simulink model "sim_all"  (R2020a)
settings: Solver=VariableStepAuto  StartTime=0.0  StopTime=2000  RelTol=1e-3
undefined symbols (not defined in the file or in its folder): a1, a2, alpha1, alpha2, cornerA, cornerB, cornerC, cornerD, ctrl_clockwise, ctrl_int_bound_or, ctrl_int_bound_pos, ctrl_k_or, ctrl_k_pos, ctrl_Ki_vel, ctrl_Kp_v_pos, ctrl_Kp_vel, ctrl_TAM, ctrl_Ts, ctrl_va_uncontrolled, ctrl_vel_uncontrolled, D, dead_zone_limit, depth, DiscIntNeverNeededParam, distanceFromWall, initInspectedSide, initPoint, mod_A, mod_Cd_F, mod_Cd_M, mod_eta_init, mod_g, mod_h0, mod_Ixx, mod_Iyy, mod_Izz, mod_Kp_dot, mod_lat0, mod_lon0, mod_m, mod_Mq_dot, mod_ni_init, mod_Nr_dot, mod_p1, mod_p2, mod_p3, mod_p4, mod_p5, mod_p6, mod_R, mod_Rm, mod_t1, mod_t2, mod_t3, mod_t4, mod_t5, mod_t6, mod_W, mod_Xu_dot, mod_Yv_dot ... (+53)
libraries: simulink x8, cstblocks x6, simulink_extras x1
(part 2 of 6)

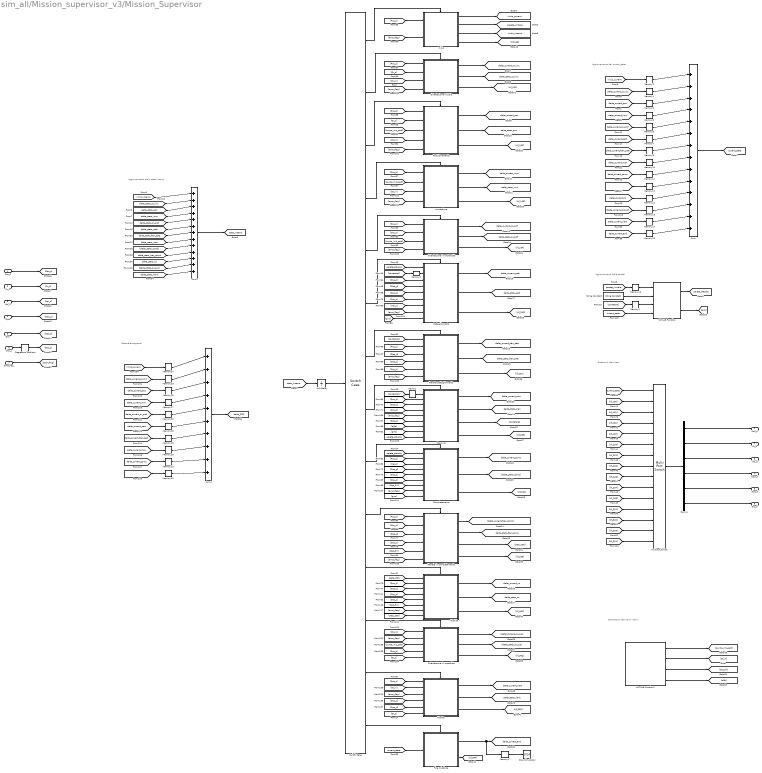
== system sim_all/Mission_supervisor_v3/Mission_Supervisor ==
  note: Gestore emergenza
  note: Generatore riferimenti interni
  note: Aggiornamento dello stato interno
  note: Aggiornamento del current_state
  note: Aggiornamento della parete
  note: Gestore di riferimenti
  Pos_S : Inport
  Or_S : Inport  Port=2
  Vel_S : Inport  Port=3
  Dpp : Inport  Port=4
  Dps : Inport  Port=5
  Orp_s : Inport  Port=6
  error_flag : Inport  Port=7
  Completamento : Subsystem  TreatAsAtomicUnit=on
  Degrees to Radians : simulink_extras/Transformations/Degrees to Radians
  Demux : Demux  Outputs=[3,3,1,1,1,1]
  Fine missione : Subsystem  TreatAsAtomicUnit=on
  Frenata in completamento : Subsystem  TreatAsAtomicUnit=on
  Frenata pattugliamento : Subsystem  TreatAsAtomicUnit=on
  Immersione : Subsystem  TreatAsAtomicUnit=on
  Inizio : Subsystem  TreatAsAtomicUnit=on
  MATLAB Function : MATLAB Function  TreatAsAtomicUnit=on
  MATLAB Function1 : MATLAB Function  TreatAsAtomicUnit=on
  Manovra : Subsystem  TreatAsAtomicUnit=on
  Memory{,1..2,4..15,17..21,25..30} (26 alike) : Memory
  Memory16 : Memory  InitialCondition=initInspectedSide
  Memory24 : Memory  InitialCondition=100
  Memory3 : Memory  InitialCondition=100
  Multiport Switch : MultiPortSwitch  DataPortOrder=Specify indices  Inputs=2  DataPortIndices={100,101,102,103,104,201,202,203,204,205,301,302,303,304}
  Orientazione Iniziale : Subsystem  TreatAsAtomicUnit=on
  Orientazione in profondità : Subsystem  TreatAsAtomicUnit=on
  Orientazione in superficie : Subsystem  TreatAsAtomicUnit=on
  Pattugliamento : Subsystem  TreatAsAtomicUnit=on
  Posizionamento : Subsystem  TreatAsAtomicUnit=on
  Rientro : Subsystem  TreatAsAtomicUnit=on
  Risalita : Subsystem  TreatAsAtomicUnit=on
  Stop Simulation : Stop
  String Constant : StringConstant  String=inspectionDirection
  Sum : Sum  Inputs=|++++++++++++++
  Sum1 : Sum  Inputs=|+++++++++++++
  Sum4 : Sum  Inputs=|++++++++++
  Switch Case : SwitchCase  CaseConditions={100,101,102,103,104,201,202,203,204,205,301,302,303,304}  ShowDefaultCase=off
  Unit Delay : UnitDelay  InitialCondition=stato  SampleTime=Ts_supervisor  HasFrameUpgradeWarning=on
  Pos_d : Outport
  Or_d : Outport  Port=2
  Vel_d : Outport  Port=3
  Dpp_d : Outport  Port=4
  Dps_d : Outport  Port=5
  Orp_d : Outport  Port=6
  tag scope: current_state=global, delta_SOS=global, delta_current_comp=global, delta_current_end=global, delta_current_fren_patt=global, delta_current_imm=global, delta_current_man=global, delta_current_or_iniz=global, delta_current_or_prof=global, delta_current_patt=global, delta_current_pos=global, delta_current_rient=global, delta_current_ris=global, delta_stato_fren_comp=global, delta_stato_fren_patt=global, delta_stato_imm=global, delta_stato_man=global, delta_stato_or_iniz=global, delta_stato_or_prof=global, delta_stato_patt=global, delta_stato_pos=global, delta_stato_rient=global, delta_stato_ris=global, inizio_current=global, inizio_interno=global, parete_attuale=global, parete_iniziale=global, stato_interno=global
  wires:
  [delta_stato_fren_comp] -> Sum1/10
  [delta_SOS] -> Risalita/1(delta_SOS)
  [delta_current_patt] -> Memory7/1
  [delta_current_pos] -> Memory5/1
  Immersione/1(delta_current_immers) -> [delta_current_imm]
  Posizionamento/3(Outport) -> [rif_102]
  Rientro/2(delta_stato_rient) -> [delta_stato_rient]
  [delta_stato_or_iniz] -> Sum1/2
  [inizio_interno] -> Sum1/1
  Memory6/1 -> Sum/4
  Orientazione Iniziale/1(delta_current_or_iniz) -> [delta_current_or_iniz]
  [delta_current_end] -> Memory15/1
  Pattugliamento/1(delta_current_patt) -> [delta_current_patt]
  Memory15/1 -> Sum/14
  Orientazione in profondità/2(delta_stato_or_prof) -> [delta_stato_or_prof]
  Memory12/1 -> Sum/10
  Memory8/1 -> Sum/7
  Completamento/3(Outport) -> [rif_204]
  Pattugliamento/2(delta_stato_patt) -> [delta_stato_patt]
  [delta_stato_man] -> Sum1/8
  Frenata in completamento/1(delta_current_fren_comp) -> [delta_current_fren_comp]
  Frenata pattugliamento/1(delta_current_fren_patt) -> [delta_current_fren_patt]
  Sum/1 -> [current_state]
  Inizio/1(current_state) -> [inizio_current]
  Memory4/1 -> Sum/2
  Posizionamento/2(delta_stato_posiz) -> [delta_stato_pos]
  [delta_stato_pos] -> Sum1/3
  Completamento/2(delta_stato_comp) -> [delta_stato_comp]
  [contatore] -> Memory2/1
  Memory17/1 -> Stop Simulation/1
  [delta_stato_imm] -> Sum1/4
  [delta_current_imm] -> Memory6/1
  [stato_interno] -> Unit Delay/1
  Sum1/1 -> [stato_interno]
  Inizio/2(parete_attuale) -> [parete_iniziale]
  [delta_stato_comp] -> Sum1/9
  [delta_stato_patt] -> Sum1/6
  Risalita/2(delta_stato_ris) -> [delta_stato_ris]
  [delta_current_fren_patt] -> Memory8/1
  [delta_current_or_prof] -> Memory9/1
  Rientro/1(delta_current_rient) -> [delta_current_rient]
  [current_state] -> Fine missione/1(current_state)
  Unit Delay/1 -> Switch Case/1
  [parete_attuale] -> Pattugliamento/1(parete)
  Memory7/1 -> Sum/6
  Orientazione in profondità/1(delta_current_or_prof) -> [delta_current_or_prof]
  Frenata in completamento/2(delta_stato_fren_comp) -> [delta_stato_fren_comp]
  [contatore] -> Frenata pattugliamento/1(contatore)
  Manovra/1(delta_current_man) -> [delta_current_man]
  [delta_current_fren_comp] -> Memory12/1
  Fine missione/1(delta_current_end) -> [delta_current_end], Memory17/1
  [inizio_current] -> Memory3/1
  [parete_attuale] -> Completamento/1(parete)
  Memory3/1 -> Sum/1
  Risalita/1(delta_current_ris) -> [delta_current_ris]
  [delta_stato_or_prof] -> Sum1/5
  Memory2/1 -> Pattugliamento/2(contatore)
  Memory11/1 -> Sum/9
  Posizionamento/1(delta_current_posiz) -> [delta_current_pos]
  Rientro/3(Outport) -> [rif_303]
  Inizio/3(delta_stato) -> [inizio_interno]
  [delta_current_comp] -> Memory11/1
  [delta_stato_fren_patt] -> Sum1/7
  [delta_stato_ris] -> Sum1/11
  Orientazione in profondità/3(Outport) -> [rif_104]
  Frenata pattugliamento/3(Outport) -> [rif_202]
  Orientazione Iniziale/2(delta_stato_or_iniz) -> [delta_stato_or_iniz]
  Fine missione/2(Outport) -> [rif_304]
  Memory10/1 -> Sum/8
  [delta_current_man] -> Memory10/1
  Immersione/2(delta_stato_immers) -> [delta_stato_imm]
  Manovra/2(delta_stato_man) -> [delta_stato_man]
  Orientazione Iniziale/3(Outport) -> [rif_101]
  [delta_current_or_iniz] -> Memory4/1
  Pattugliamento/3(Outport) -> [rif_201]
  Frenata pattugliamento/2(delta_stato_fren_patt) -> [delta_stato_fren_patt]
  Memory9/1 -> Sum/5
  Memory14/1 -> Sum/13
  Inizio/4(Outport) -> [rif_100]
  Risalita/3(Outport) -> [rif_301]
  Immersione/3(Outport) -> [rif_103]
  Memory5/1 -> Sum/3
  [Pos_s] -> Inizio/1(Pos_s)
  [Pos_s] -> Orientazione Iniziale/1(Pos_s)
  [Pos_s] -> Posizionamento/1(Pos_s)
  [Pos_s] -> Immersione/1(Pos_s)
  [Pos_s] -> Frenata pattugliamento/2(Pos_s)
  [Dpp_s] -> Frenata pattugliamento/3(Dpp_s)
  [Dps_s] -> Frenata pattugliamento/4(Dps_s)
  [Pos_s] -> Pattugliamento/3(Pos_s)
  [Dpp_s] -> Pattugliamento/4(Dpp_s)
  [Dps_s] -> Pattugliamento/5(Dps_s)
  [Orp_s] -> Pattugliamento/6(Orp_s)
  [Vel_s] -> Pattugliamento/7(Vel_s)
  [Orp_s] -> Frenata pattugliamento/5(Orp_s)
  [Dpp_s] -> Manovra/3(Dpp_s)
  [Orp_s] -> Manovra/4(Orp_s)
  [Pos_s] -> Manovra/2(Pos_s)
  [Pos_s] -> Completamento/2(Pos_s)
  [Vel_s] -> Completamento/3(Vel_s)
  [Dpp_s] -> Completamento/4(Dpp_s)
  [Dps_s] -> Completamento/5(Dps_s)
  [Orp_s] -> Completamento/6(Orp_s)
  [Pos_s] -> Frenata in completamento/1(Pos_s)
  [Orp_s] -> Frenata in completamento/2(Orp_s)
  [Dpp_s] -> Frenata in completamento/3(Dpp_s)
  [Dps_s] -> Frenata in completamento/4(Dps_s)
  [Pos_s] -> Risalita/2(Pos_s)
  [Dpp_s] -> Risalita/3(Dpp_s)
  [Pos_s] -> Rientro/1(Pos_s)
  Demux/2 -> Or_d/1
  [rif_202] -> Multiport Switch/8
  [current_state] -> Multiport Switch/1
  Demux/6 -> Orp_d/1
  Demux/3 -> Vel_d/1
  Multiport Switch/1 -> Demux/1
  [rif_301] -> Multiport Switch/12
  Demux/4 -> Dpp_d/1
  [rif_102] -> Multiport Switch/4
  [rif_203] -> Multiport Switch/9
  Demux/5 -> Dps_d/1
  Demux/1 -> Pos_d/1
  [rif_302] -> Multiport Switch/13
  [rif_201] -> Multiport Switch/7
  [rif_104] -> Multiport Switch/6
  [rif_205] -> Multiport Switch/11
  [rif_204] -> Multiport Switch/10
  [rif_101] -> Multiport Switch/3
  [rif_303] -> Multiport Switch/14
  [rif_103] -> Multiport Switch/5
  Completamento/1(delta_current_comp) -> [delta_current_comp]
  [Pos_s] -> Orientazione in profondità/1(Pos_s)
  [Orp_s] -> Orientazione in profondità/2(Orp_s)
  [rif_100] -> Multiport Switch/2
  [Or_s] -> Orientazione Iniziale/2(Or_s)
  [Or_in] -> Orientazione Iniziale/3(Or_in)
  [Or_in] -> Posizionamento/4(Or_in)
  [punto_iniz_patt] -> Posizionamento/3(punto iniziale)
  [dps_fin] -> Frenata in completamento/5(dps_fin)
  [punto_iniz_patt] -> Immersione/2(punto_iniz_patt)
  [punto_iniz_patt] -> Orientazione in profondità/3(Punto_iniz_patt)
  [Or_s] -> Posizionamento/2(Or_s)
  [dps_fin] -> Completamento/7(Dps_fin)
  error_flag/1 -> [error_flag]
  [error_flag] -> Frenata in completamento/6(error_flag)
  [error_flag] -> Completamento/8(error_flag)
  [error_flag] -> Manovra/5(error_flag)
  [error_flag] -> Frenata pattugliamento/6(error_flag)
  [error_flag] -> Pattugliamento/8(error_flag)
  [error_flag] -> Orientazione in profondità/4(error_flag)
  [error_flag] -> Immersione/4(error_flag)
  [error_flag] -> Posizionamento/5(error_flag)
  [error_flag] -> Orientazione Iniziale/4(error_flag)
  [error_flag] -> Inizio/2(error_flag)
  MATLAB Function1/3(dps_fin) -> [dps_fin]
  MATLAB Function1/2(Or_in) -> [Or_in]
  MATLAB Function1/1(punto_iniz_patt) -> [punto_iniz_patt]
  [Or_in] -> Immersione/3(Or_in)
  [Or_in] -> Rientro/2(Or_in)
  Memory25/1 -> Sum4/2
  Sum4/1 -> [delta_SOS]
  Memory27/1 -> Sum4/4
  Memory20/1 -> Sum4/10
  [delta_current_fren_comp] -> Memory20/1
  Memory26/1 -> Sum4/3
  Memory28/1 -> Sum4/6
  [delta_current_comp] -> Memory19/1
  Memory18/1 -> Sum4/8
  [delta_current_or_prof] -> Memory30/1
  Memory30/1 -> Sum4/5
  [delta_current_or_iniz] -> Memory25/1
  [delta_current_man] -> Memory18/1
  [delta_current_fren_patt] -> Memory29/1
  [delta_current_patt] -> Memory28/1
  [inizio_current] -> Memory24/1
  [delta_current_pos] -> Memory26/1
  [delta_current_imm] -> Memory27/1
  Memory24/1 -> Sum4/1
  Memory29/1 -> Sum4/7
  Memory19/1 -> Sum4/9
  [contatore] -> Memory1/1
  [parete_iniziale] -> Memory16/1
  [current_state] -> MATLAB Function/4(current_state)
  Memory1/1 -> MATLAB Function/3(contatore)
  String Constant/1 -> MATLAB Function/2(verso)
  Memory16/1 -> MATLAB Function/1(parete_iniziale)
  MATLAB Function/1(parete) -> [parete_attuale]
  [contatore] -> Memory/1
  Memory/1 -> Manovra/1(contatore)
  [Dps_s] -> Risalita/5(Dps_s)
  [Orp_s] -> Risalita/4(Orp_s)
  [dps_fin] -> Risalita/6(Dps_fin)
  Switch Case/1 -> Inizio/Action
  Switch Case/3 -> Posizionamento/Action
  Switch Case/2 -> Orientazione Iniziale/Action
  Switch Case/4 -> Immersione/Action
  Switch Case/5 -> Orientazione in profondità/Action
  Switch Case/6 -> Pattugliamento/Action
  Switch Case/7 -> Frenata pattugliamento/Action
  Switch Case/8 -> Manovra/Action
  Switch Case/9 -> Completamento/Action
  Switch Case/10 -> Frenata in completamento/Action
  Switch Case/11 -> Risalita/Action
  Switch Case/12 -> Orientazione in superficie/Action
  Switch Case/13 -> Rientro/Action
  Switch Case/14 -> Fine missione/Action
  Orientazione in superficie/1(delta_current_or_sup) -> [delta_current_or_sup]
  Orientazione in superficie/2(delta_stato_or_sup) -> [delta_stato_or_sup]
  Orientazione in superficie/3(Outport) -> [rif_302]
  [rif_304] -> Multiport Switch/15
  [error_flag] -> Risalita/7(error_flag)
  Memory13/1 -> Sum/12
  Memory21/1 -> Sum/11
  [delta_stato_or_sup] -> Sum1/12
  [delta_stato_rient] -> Sum1/13
  [delta_current_rient] -> Memory14/1
  [delta_current_or_sup] -> Memory13/1
  [delta_current_ris] -> Memory21/1
  [error_flag] -> Rientro/3(error_flag)
  [error_flag] -> Orientazione in superficie/2(error_flag)
  [Or_in] -> Orientazione in superficie/1(Or_in)
  [punto_iniz_patt] -> Orientazione in superficie/3(punto_iniz_patt)
  [Or_s] -> Orientazione in superficie/5(Or_s)
  [Pos_s] -> Orientazione in superficie/4(Pos_s)
  [Dps_s] -> Rientro/4(Dps_s)
  [Dpp_s] -> Rientro/5(Dpp_s)
  [Dps_s] -> Manovra/6(Dps_s)
  MATLAB Function/2(giro) -> [giro]
  [giro] -> Pattugliamento/9(giro)
  [giro] -> Completamento/9(giro)
  [SOS_205] -> Risalita/8(SOS_205)
  Pos_S/1 -> [Pos_s]
  Or_S/1 -> [Or_s]
  Vel_S/1 -> [Vel_s]
  Dpp/1 -> [Dpp_s]
  Dps/1 -> [Dps_s]
  Orp_s/1 -> Degrees to Radians/1
  Degrees to Radians/1 -> [Orp_s]
  Manovra/4("  ") -> [rif_203]
  Manovra/3(contatore_out) -> [contatore]
  Frenata in completamento/3(SOS_205) -> [SOS_205]
  Frenata in completamento/4(" ") -> [rif_205]
  [Or_s] -> Rientro/6(Or_s)
  MATLAB Function1/4(alfa) -> [alfa]
  [alfa] -> Manovra/7(alfa)
  [giro] -> Manovra/8(giro)
  [parete_attuale] -> Manovra/9(parete_attuale)

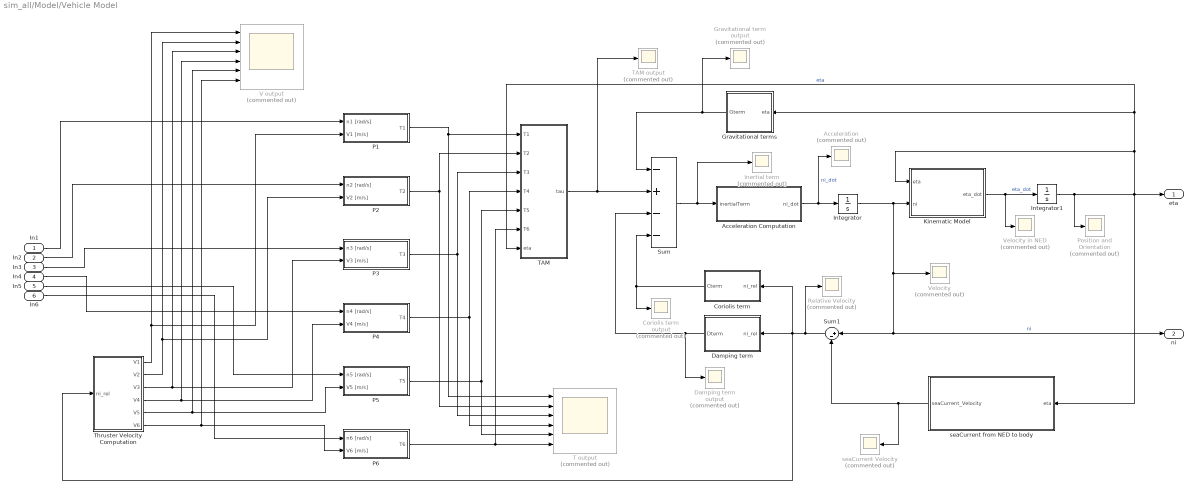
== system sim_all/Model/Vehicle Model ==
  In1 : Inport
  In2 : Inport  Port=2
  In3 : Inport  Port=3
  In4 : Inport  Port=4
  In5 : Inport  Port=5
  In6 : Inport  Port=6
  Acceleration : Scope  Commented=on
  Acceleration Computation : MATLAB Function  TreatAsAtomicUnit=on
  Coriolis term : MATLAB Function  TreatAsAtomicUnit=on
  Coriolis term output : Scope  Commented=on
  Damping term : MATLAB Function  TreatAsAtomicUnit=on
  Damping term output : Scope  Commented=on
  Gravitational term output : Scope  Commented=on
  Gravitational terms : MATLAB Function  TreatAsAtomicUnit=on
  Inertial term : Scope  Commented=on
  Integrator : Integrator  InitialCondition=mod_ni_init
  Integrator1 : Integrator  InitialCondition=mod_eta_init
  Kinematic Model : MATLAB Function  TreatAsAtomicUnit=on
  P1 : Subsystem
  P2 : Subsystem
  P3 : Subsystem
  P4 : Subsystem
  P5 : Subsystem
  P6 : Subsystem
  Position and Orientation : Scope  Commented=on
  Relative Velocity : Scope  Commented=on
  Sum : Sum  Inputs=-+--
  Sum1 : Sum  Inputs=|+-
  T output : Scope  Commented=on  NumInputPorts=6
  TAM : MATLAB Function  TreatAsAtomicUnit=on
  TAM output : Scope  Commented=on
  Thruster Velocity Computation : MATLAB Function  TreatAsAtomicUnit=on
  V output : Scope  Commented=on  NumInputPorts=6
  Velocity : Scope  Commented=on
  Velocity in NED : Scope  Commented=on
  seaCurrent Velocity : Scope  Commented=on
  seaCurrent from NED to body : MATLAB Function  TreatAsAtomicUnit=on
  eta : Outport
  ni : Outport  Port=2
  wires:
  P3/1(T3) -> TAM/3(T3), T output/3
  P5/1(T5) -> TAM/5(T5), T output/5
  P6/1(T6) -> TAM/6(T6), T output/6
  Thruster Velocity Computation/6(V6) -> P6/2(V6 [m/s]), V output/6
  Sum/1 -> Acceleration Computation/1(inertialTerm), Inertial term/1
  Integrator/1 -> Kinematic Model/2(ni), Velocity/1, ni/1, Sum1/1  "ni"
  P2/1(T2) -> TAM/2(T2), T output/2
  Acceleration Computation/1(ni_dot) -> Integrator/1, Acceleration/1  "ni_dot"
  Gravitational terms/1(Gterm) -> Sum/1, Gravitational term output/1
  P1/1(T1) -> T output/1, TAM/1(T1)
  TAM/1(tau) -> Sum/2, TAM output/1
  Thruster Velocity Computation/5(V5) -> P5/2(V5 [m/s]), V output/5
  Integrator1/1 -> Position and Orientation/1, Kinematic Model/1(eta), Gravitational terms/1(eta), TAM/7(eta), seaCurrent from NED to body/1(eta), eta/1  "eta"
  Thruster Velocity Computation/2(V2) -> V output/2, P2/2(V2 [m/s])
  Thruster Velocity Computation/1(V1) -> V output/1, P1/2(V1 [m/s])
  Damping term/1(Dterm) -> Damping term output/1, Sum/3
  Kinematic Model/1(eta_dot) -> Integrator1/1, Velocity in NED/1  "eta_dot"
  P4/1(T4) -> TAM/4(T4), T output/4
  Thruster Velocity Computation/4(V4) -> P4/2(V4 [m/s]), V output/4
  Thruster Velocity Computation/3(V3) -> P3/2(V3 [m/s]), V output/3
  Coriolis term/1(Cterm) -> Coriolis term output/1, Sum/4
  In6/1 -> P6/1(n6 [rad/s])
  In2/1 -> P2/1(n2 [rad/s])
  In5/1 -> P5/1(n5 [rad/s])
  In1/1 -> P1/1(n1 [rad/s])
  In4/1 -> P4/1(n4 [rad/s])
  In3/1 -> P3/1(n3 [rad/s])
  seaCurrent from NED to body/1(seaCurrent_Velocity) -> seaCurrent Velocity/1, Sum1/2
  Sum1/1 -> Relative Velocity/1, Thruster Velocity Computation/1(ni_rel), Damping term/1(ni_rel), Coriolis term/1(ni_rel)

== system sim_all/Navigation/Calcolo distaza pareti ==
  orient : Inport
  pos_es : Inport  Port=2
  Calcolo distanza dalle pareti : MATLAB Function  TreatAsAtomicUnit=on
  Calcolo orientazione dalla parete : MATLAB Function  TreatAsAtomicUnit=on
  dpp : Outport
  dps : Outport  Port=2
  orient_parete : Outport  Port=3
  wires:
  pos_es/1 -> Calcolo distanza dalle pareti/1(pos_es), Calcolo orientazione dalla parete/1(pos_es)
  Calcolo distanza dalle pareti/2(dps) -> dps/1
  Calcolo orientazione dalla parete/1(orient_parete) -> orient_parete/1
  orient/1 -> Calcolo orientazione dalla parete/3(orient)
  Calcolo distanza dalle pareti/1(dpp) -> dpp/1
  [parete_attuale] -> Calcolo distanza dalle pareti/2(parete_attuale), Calcolo orientazione dalla parete/2(parete_attuale)

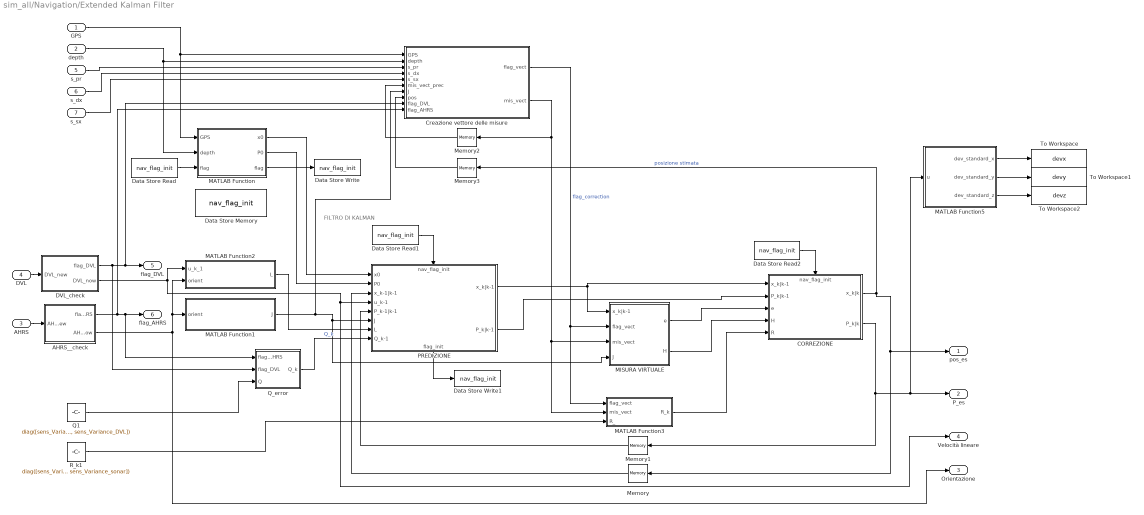
== system sim_all/Navigation/Extended Kalman Filter ==
  note: FILTRO DI KALMAN
  GPS : Inport
  depth : Inport  Port=2
  AHRS : Inport  Port=3
  DVL : Inport  Port=4
  s_pr : Inport  Port=5
  s_dx : Inport  Port=6
  s_sx : Inport  Port=7
  AHRS__check : Subsystem
  CORREZIONE : Subsystem
      settings: PortSchema="{\"entries\":[{\"content\":{\"sides\":[{\"content\":{\"connectorIds\":[\"In1\",\"In2\",\"In3\",\"In4\",\"In5\"]},\"type\":\"ConnectorPlacement.EquallySpacedRectSide\",\"uuid\":\"44d4b6e6-a4db-4e12-b0bf-41ec8347b107\"},{\"content\":{\"connectorIds\":[\"Out1\",\"Out2\"],\"side\":\"RIGHT\"},\"type\":\"ConnectorPlacement.EquallySpacedRectSide\",\"uuid\":\"9e6d7b97-2a84-49ec-a092-e75c60e4106f\"},{\"content\":{\"connectorIds\":[\"In6\"],\"side\":\"TOP\"},\"type\":\"ConnectorPlacement.EquallySpacedRectSide\",\"uuid\":\"c5d17fe6-9815-494d-a6f8-5d09015b4aeb\"}]},\"type\":\"ConnectorPlacement.EquallySpacedConnector\",\"uuid\":\"e87b91ff-8818-4035-b847-a1a4860b11e5\"}],\"packageUris\":[\"http://schema.mathworks.com/mf0/Connector/19700101\"],\"version\":\"1.0\"}"
  Creazione vettore delle misure : MATLAB Function  TreatAsAtomicUnit=on  SystemSampleTime=nav_DT
  DVL_check : Subsystem
  Data Store Memory : DataStoreMemory  DataStoreName=nav_flag_init  ShowAdditionalParam=off
  Data Store Read : DataStoreRead  DataStoreName=nav_flag_init  DataStoreElements=nav_flag_init
  Data Store Read1 : DataStoreRead  DataStoreName=nav_flag_init  DataStoreElements=nav_flag_init
  Data Store Read2 : DataStoreRead  DataStoreName=nav_flag_init  DataStoreElements=nav_flag_init
  Data Store Write : DataStoreWrite  DataStoreName=nav_flag_init  DataStoreElements=nav_flag_init
  Data Store Write1 : DataStoreWrite  DataStoreName=nav_flag_init  DataStoreElements=nav_flag_init
  MATLAB Function : MATLAB Function  TreatAsAtomicUnit=on
  MATLAB Function1 : MATLAB Function  TreatAsAtomicUnit=on
  MATLAB Function2 : MATLAB Function  TreatAsAtomicUnit=on
  MATLAB Function3 : MATLAB Function  TreatAsAtomicUnit=on  SystemSampleTime=nav_DT
  MATLAB Function5 : MATLAB Function  TreatAsAtomicUnit=on
  MISURA VIRTUALE : Subsystem
  Memory{,1..3} (4 alike) : Memory
  PREDIZIONE : Subsystem
      settings: PortSchema="{\"entries\":[{\"content\":{\"sides\":[{\"content\":{\"connectorIds\":[\"In1\",\"In2\",\"In3\",\"In4\",\"In5\",\"In6\",\"In7\",\"In8\"]},\"type\":\"ConnectorPlacement.EquallySpacedRectSide\",\"uuid\":\"afcfc03b-4c18-49df-ab20-1356d76b0e63\"},{\"content\":{\"connectorIds\":[\"Out1\",\"Out2\"],\"side\":\"RIGHT\"},\"type\":\"ConnectorPlacement.EquallySpacedRectSide\",\"uuid\":\"f068ce64-2e14-41bc-9570-b9ba38e252ee\"},{\"content\":{\"connectorIds\":[\"In9\"],\"side\":\"TOP\"},\"type\":\"ConnectorPlacement.EquallySpacedRectSide\",\"uuid\":\"07751979-165e-45fb-8dea-4cc1ad3e58f3\"},{\"content\":{\"connectorIds\":[\"Out3\"],\"side\":\"BOTTOM\"},\"type\":\"ConnectorPlacement.EquallySpacedRectSide\",\"uuid\":\"3c36a795-b00b-49e7-8b71-9706a2c2134a\"}]},\"type\":\"ConnectorPlacement.EquallySpacedConnector\",\"uuid\":\"bde89349-47ff-4cbc-a848-02c48716c9c8\"}],\"packageUris\":[\"http://schema.mathworks.com/mf0/Connector/19700101\"],\"version\":\"1.0\"}"
  Q1 : Constant  Value=diag([sens_Variance_AHRS_roll, sens_Variance_AHRS_pitch, sens_Variance_AHRS_yaw, sens_Variance_DVL, sens_Variance_DVL, sens_Variance_DVL])  VectorParams1D=off
  Q_error : Subsystem
  R_k1 : Constant  Value=diag([sens_Variance_GPS, sens_Variance_GPS, sens_Variance_depth1, sens_Variance_sonar, sens_Variance_sonar, sens_Variance_sonar])  VectorParams1D=off
  To Workspace : ToWorkspace  VariableName=devx  SaveFormat=Timeseries  SampleTime=-1
  To Workspace1 : ToWorkspace  VariableName=devy  SaveFormat=Timeseries  SampleTime=-1
  To Workspace2 : ToWorkspace  VariableName=devz  SaveFormat=Timeseries  SampleTime=-1
  pos_es : Outport
  P_es : Outport  Port=2
  Orientazione : Outport  Port=3
  Velocità lineare : Outport  Port=4
  flag_DVL : Outport  Port=5
  flag_AHRS : Outport  Port=6
  wires:
  PREDIZIONE/1(x_k|k-1) -> CORREZIONE/1(x_k|k-1), MISURA VIRTUALE/1(x_k|k-1)
  PREDIZIONE/2(P_k|k-1) -> CORREZIONE/2(P_k|k-1)
  Memory/1 -> PREDIZIONE/3(x_k-1|k-1)
  CORREZIONE/2(P_k|k) -> Memory1/1, P_es/1, MATLAB Function5/1(u)
  Memory1/1 -> PREDIZIONE/5(P_k-1|k-1)
  MISURA VIRTUALE/2(H) -> CORREZIONE/4(H)
  MISURA VIRTUALE/1(e) -> CORREZIONE/3(e)
  GPS/1 -> MATLAB Function/1(GPS), Creazione vettore delle misure/1(GPS)
  depth/1 -> MATLAB Function/2(depth), Creazione vettore delle misure/2(depth)
  s_pr/1 -> Creazione vettore delle misure/3(s_pr)
  Creazione vettore delle misure/2(mis_vect) -> MATLAB Function3/2(mis_vect), MISURA VIRTUALE/3(mis_vect), Memory2/1
  Memory2/1 -> Creazione vettore delle misure/6(mis_vect_prec)
  Creazione vettore delle misure/1(flag_vect) -> MATLAB Function3/1(flag_vect), MISURA VIRTUALE/2(flag_vect)  "flag_correction"
  s_dx/1 -> Creazione vettore delle misure/4(s_dx)
  s_sx/1 -> Creazione vettore delle misure/5(s_sx)
  MATLAB Function/2(P0) -> PREDIZIONE/2(P0)
  MATLAB Function/1(x0) -> PREDIZIONE/1(x0)
  MATLAB Function1/1(J) -> Creazione vettore delle misure/7(J), MISURA VIRTUALE/4(J), PREDIZIONE/6(J)
  MATLAB Function2/1(L) -> PREDIZIONE/7(L)
  Data Store Read/1 -> MATLAB Function/3("flag ")
  MATLAB Function/3(flag) -> Data Store Write/1
  Data Store Read1/1 -> PREDIZIONE/9(nav_flag_init)
  Data Store Read2/1 -> CORREZIONE/6(nav_flag_init)
  PREDIZIONE/3(flag_init) -> Data Store Write1/1
  R_k1/1 -> MATLAB Function3/3(R_)
  MATLAB Function3/1(R_k) -> CORREZIONE/5(R)
  CORREZIONE/1(x_k|k) -> pos_es/1, Memory/1, Memory3/1  "posizione stimata"
  Memory3/1 -> Creazione vettore delle misure/8(pos)
  AHRS__check/2(AHRS_now) -> Orientazione/1, MATLAB Function2/2(orient), MATLAB Function1/1(orient)
  DVL_check/2(DVL_now) -> Velocità lineare/1, PREDIZIONE/4(u_k-1), MATLAB Function2/1(u_k_1)
  DVL/1 -> DVL_check/1(DVL_new)
  AHRS/1 -> AHRS__check/1(AHRS_new)
  DVL_check/1(flag_DVL) -> flag_DVL/1, Creazione vettore delle misure/9(flag_DVL), Q_error/2(flag_DVL)
  AHRS__check/1(flag_AHRS) -> flag_AHRS/1, Q_error/1(flag_AHRS), Creazione vettore delle misure/10(flag_AHRS)
  Q1/1 -> Q_error/3(Q)
  Q_error/1(Q_k) -> PREDIZIONE/8(Q_k-1)  "Q_k"
  MATLAB Function5/1(dev_standard_x) -> To Workspace/1
  MATLAB Function5/2(dev_standard_y) -> To Workspace1/1
  MATLAB Function5/3(dev_standard_z) -> To Workspace2/1

== system sim_all/Navigation/Filtro AHRS ==
  AHRS : Inport
  Filtro 1 : DiscreteFir  Coefficients=[0.2 0.2 0.2 0.1 0.1 0.1 0.1]  SampleTime=0.1
  Orientazione : Outport
  wires:
  AHRS/1 -> Filtro 1/1
  Filtro 1/1 -> Orientazione/1

== system sim_all/Navigation/Filtro DVL ==
  DVL : Inport
  Demux : Demux  Outputs=3
  Filtro 2 : DiscreteFir  Coefficients=[0.3 0.3 0.2 0.2]  SampleTime=0.1
  Filtro 3 : DiscreteFir  Coefficients=[0.3 0.3 0.2 0.2]  SampleTime=0.1
  Mux : Mux  Inputs=3
  Velocità lineare : Outport
  wires:
  Filtro 2/1 -> Mux/1
  Demux/3 -> Mux/3
  DVL/1 -> Demux/1
  Filtro 3/1 -> Mux/2
  Mux/1 -> Velocità lineare/1  "DVL"
  Demux/1 -> Filtro 2/1
  Demux/2 -> Filtro 3/1

== system sim_all/Navigation/Filtro Gyro ==
  Gyro : Inport
  Filtro 1 : DiscreteFir  Coefficients=[0.9 0.05 0.05]  SampleTime=0.1
  Velocità Angolare : Outport
  wires:
  Gyro/1 -> Filtro 1/1
  Filtro 1/1 -> Velocità Angolare/1

== system sim_all/Navigation/Gyro_check ==
  Gyro_new : Inport
  MATLAB Function4 : MATLAB Function  TreatAsAtomicUnit=on
  Memory4 : Memory
  flag_Gyro : Outport
  Gyro_now : Outport  Port=2
  wires:
  Gyro_new/1 -> MATLAB Function4/1(gyro_new)
  Memory4/1 -> MATLAB Function4/2(gyro_old)
  MATLAB Function4/1(flag_gyro) -> flag_Gyro/1
  MATLAB Function4/2(gyro_now) -> Memory4/1, Gyro_now/1

== system sim_all/Navigation/SOS_flag_generator ==
  P_es : Inport
  AHRS : Inport  Port=2
  DVL : Inport  Port=3
  Gyro : Inport  Port=4
  MATLAB Function : MATLAB Function  TreatAsAtomicUnit=on  SystemSampleTime=nav_DT
  Memory : Memory
  nav_SOS : Outport
  tag scope: nav_contatore=global
  wires:
  MATLAB Function/1(SOS) -> nav_SOS/1
  AHRS/1 -> MATLAB Function/3(AHRS)
  DVL/1 -> MATLAB Function/2(DVL)
  P_es/1 -> MATLAB Function/1(P_es)
  [nav_contatore] -> Memory/1
  MATLAB Function/2(contatore) -> [nav_contatore]
  Gyro/1 -> MATLAB Function/4(gyro)
  Memory/1 -> MATLAB Function/5("contatore ")

== system sim_all/Sensors/BLOCCO AHRS1 ==
  note: R  [rad]
      | P  [rad]
  note: Y [rad]
  orient_real : Inport  SampleTime=sens_Sample_time_AHRS
  orient_real1 : Inport  Port=2  SampleTime=sens_Sample_time_AHRS
  orient_real2 : Inport  Port=3  SampleTime=sens_Sample_time_AHRS
  Mux2 : Mux  Inputs=2
  Quantizer : Quantizer  QuantizationInterval=sens_Resolution_AHRS  LinearizeAsGain=off
  Quantizer1 : Quantizer  QuantizationInterval=sens_Resolution_AHRS  LinearizeAsGain=off
  Quantizer2 : Quantizer  QuantizationInterval=sens_Resolution_AHRS  LinearizeAsGain=off
  Random Number : RandomNumber  Variance=sens_Variance_AHRS_roll  Seed=5678  SampleTime=sens_Sample_time_AHRS
  Random Number1 : RandomNumber  Variance=sens_Variance_AHRS_pitch  Seed=4562  SampleTime=sens_Sample_time_AHRS
  Random Number2 : RandomNumber  Variance=sens_Variance_AHRS_yaw  Seed=1258  SampleTime=sens_Sample_time_AHRS
  Sum1 : Sum  Inputs=|++
  Sum2 : Sum  Inputs=++|
  Sum6 : Sum  Inputs=|++
  R-P NED : Outport
  Y NED : Outport  Port=2
  wires:
  orient_real2/1 -> Sum6/1
  orient_real/1 -> Sum2/2
  Sum6/1 -> Quantizer2/1
  Mux2/1 -> R-P NED/1
  Sum2/1 -> Quantizer/1
  orient_real1/1 -> Sum1/1
  Random Number1/1 -> Sum1/2
  Sum1/1 -> Quantizer1/1
  Random Number/1 -> Sum2/1
  Random Number2/1 -> Sum6/2
  Quantizer/1 -> Mux2/1
  Quantizer1/1 -> Mux2/2
  Quantizer2/1 -> Y NED/1

== system sim_all/Sensors/BLOCCO DVL1 ==
  "DVL vx " : Inport  SampleTime=sens_Sample_time_dvl
  DVL vy : Inport  Port=2  SampleTime=sens_Sample_time_dvl
  DVL vz : Inport  Port=3  SampleTime=sens_Sample_time_dvl
  " WNoise DVL x " : RandomNumber  Variance=sens_Variance_DVL  Seed=1234  SampleTime=sens_Sample_time_dvl
  Quantizer : Quantizer  QuantizationInterval=sens_Resolution_dvl  LinearizeAsGain=off
  Quantizer1 : Quantizer  QuantizationInterval=sens_Resolution_dvl  LinearizeAsGain=off
  Quantizer2 : Quantizer  QuantizationInterval=sens_Resolution_dvl  LinearizeAsGain=off
  Sum1 : Sum  Inputs=|++
  Sum2 : Sum  Inputs=|++
  Sum3 : Sum  Inputs=|++
  WNoise DVL y : RandomNumber  Variance=sens_Variance_DVL  Seed=1235  SampleTime=sens_Sample_time_dvl
  WNoise DVL z : RandomNumber  Variance=sens_Variance_DVL  Seed=1237  SampleTime=sens_Sample_time_dvl
  DVL vx BODY : Outport
  DVL vy BODY : Outport  Port=2
  DVL vz BODY : Outport  Port=3
  wires:
  " WNoise DVL x "/1 -> Sum2/2
  Sum2/1 -> Quantizer/1
  WNoise DVL y/1 -> Sum1/2
  Sum1/1 -> Quantizer1/1
  WNoise DVL z/1 -> Sum3/2
  Sum3/1 -> Quantizer2/1
  "DVL vx "/1 -> Sum2/1
  DVL vy/1 -> Sum1/1
  DVL vz/1 -> Sum3/1
  Quantizer/1 -> DVL vx BODY/1
  Quantizer1/1 -> DVL vy BODY/1
  Quantizer2/1 -> DVL vz BODY/1

== system sim_all/Sensors/BLOCCO GPS1 ==
  note: Controllo per antenna
  "LAT " : Inport  SampleTime=sens_Sample_time_GPS
  "LON " : Inport  Port=2  SampleTime=sens_Sample_time_GPS
  DEP : Inport  Port=3  SampleTime=sens_Sample_time_GPS
  Compare To Constant : simulink/Logic and Bit Operations/Compare To Constant  relop=<  const=sens_threshold  OutDataTypeStr=uint8
  Quantizer : Quantizer  QuantizationInterval=sens_Resolution_GPS
  Quantizer1 : Quantizer  QuantizationInterval=sens_Resolution_GPS  LinearizeAsGain=off
  Sum2 : Sum  Inputs=++|
  Sum3 : Sum  Inputs=|++
  WN LAT : RandomNumber  Variance=sens_Variance_GPS  Seed=8765  SampleTime=sens_Sample_time_GPS
  WN LON : RandomNumber  Variance=sens_Variance_GPS  Seed=9876  SampleTime=sens_Sample_time_GPS
  "GPS LAT " : Outport
  "GPS LON " : Outport  Port=2
  FLAG : Outport  Port=3
  wires:
  Sum3/1 -> Quantizer/1
  "LON "/1 -> Sum3/1
  WN LON/1 -> Sum3/2
  Sum2/1 -> Quantizer1/1
  Compare To Constant/1 -> FLAG/1
  DEP/1 -> Compare To Constant/1
  WN LAT/1 -> Sum2/1
  "LAT "/1 -> Sum2/2
  Quantizer1/1 -> "GPS LAT "/1
  Quantizer/1 -> "GPS LON "/1

== system sim_all/Sensors/BLOCCO GYRO1 ==
  angvel_rea1l : Inport  SampleTime=sens_Sample_time_GYRO
  angvel_real2 : Inport  Port=2  SampleTime=sens_Sample_time_GYRO
  angvel_real3 : Inport  Port=3  SampleTime=sens_Sample_time_GYRO
  Clock1 : Clock
  Quantizer : Quantizer  QuantizationInterval=sens_Resolution_GYRO  LinearizeAsGain=off
  Quantizer1 : Quantizer  QuantizationInterval=sens_Resolution_GYRO  LinearizeAsGain=off
  Quantizer2 : Quantizer  QuantizationInterval=sens_Resolution_GYRO  LinearizeAsGain=off
  Subsystem : Subsystem
  Sum1 : Sum  Inputs=+++
  Sum2 : Sum  Inputs=+++
  Sum5 : Sum  Inputs=+++
  WN Gyro P : RandomNumber  Variance=sens_Variance_GYRO  Seed=2347  SampleTime=sens_Sample_time_GYRO
  WN Gyro R : RandomNumber  Variance=sens_Variance_GYRO  Seed=2346  SampleTime=sens_Sample_time_GYRO
  WN Gyro Y : RandomNumber  Variance=sens_Variance_GYRO  Seed=2348  SampleTime=sens_Sample_time_GYRO
  Gyro R BODY : Outport
  Gyro P BODY : Outport  Port=2
  Gyro Y BODY : Outport  Port=3
  wires:
  Sum5/1 -> Quantizer/1
  Sum1/1 -> Quantizer1/1
  Sum2/1 -> Quantizer2/1
  Quantizer/1 -> Gyro R BODY/1
  Quantizer1/1 -> Gyro P BODY/1
  Quantizer2/1 -> Gyro Y BODY/1
  angvel_rea1l/1 -> Sum5/2
  angvel_real2/1 -> Sum1/2
  WN Gyro P/1 -> Sum1/3
  angvel_real3/1 -> Sum2/2
  WN Gyro Y/1 -> Sum2/3
  Clock1/1 -> Subsystem/1(t)
  Subsystem/1(Bias_G) -> Sum2/1, Sum1/1, Sum5/1
  WN Gyro R/1 -> Sum5/3

== system sim_all/Sensors/BLOCCO PROF.1 ==
  note: [m]
  DEP : Inport  SampleTime=sens_Sample_time_depth
  Compare To Constant1 : simulink/Logic and Bit Operations/Compare To Constant  relop=<  const=50  OutDataTypeStr=boolean
  Quantizer : Quantizer  QuantizationInterval=sens_Resolution_depth  LinearizeAsGain=off
  Sum3 : Sum  Inputs=++|
  Switch : Switch  Criteria=u2 > Threshold
  "WN Prof. h< 50 " : RandomNumber  Variance=sens_Variance_depth1  Seed=6543  SampleTime=sens_Sample_time_depth
  WN Prof. h>50 : RandomNumber  Variance=sens_Variance_depth2  Seed=3210  SampleTime=sens_Sample_time_depth
  Profondimetro : Outport
  wires:
  DEP/1 -> Sum3/2, Compare To Constant1/1
  Compare To Constant1/1 -> Switch/2
  "WN Prof. h< 50 "/1 -> Switch/1
  WN Prof. h>50/1 -> Switch/3
  Switch/1 -> Sum3/1
  Sum3/1 -> Quantizer/1
  Quantizer/1 -> Profondimetro/1

== system sim_all/Sensors/Environment and Sensors Model3 ==
  LAT-LON : Inport  SampleTime=sens_Sample_time_sonar
  Environment : Inport  Port=2  SampleTime=sens_Sample_time_sonar
  AHRS Roll : Inport  Port=3  SampleTime=sens_Sample_time_sonar
  AHRS Pitch : Inport  Port=4  SampleTime=sens_Sample_time_sonar
  AHRS Yaw : Inport  Port=5  SampleTime=sens_Sample_time_sonar
  " WN Sonar DX " : RandomNumber  Variance=sens_Variance_sonar  Seed=4325  SampleTime=sens_Sample_time_sonar
  Constant : Constant  Value=sens_distCM
  Demux3 : Demux  Outputs=5
  MATLAB Function1 : MATLAB Function  TreatAsAtomicUnit=on
  Quantizer : Quantizer  QuantizationInterval=sens_Resolution_sonar  LinearizeAsGain=off
  Sum1 : Sum  Inputs=|+-
  Sum2 : Sum  Inputs=|++
  Sonar DX : Outport
  wires:
  MATLAB Function1/1(dist) -> Sum1/1
  Sum1/1 -> Sum2/1
  Constant/1 -> Sum1/2
  Environment/1 -> Demux3/1
  Quantizer/1 -> Sonar DX/1
  Demux3/4 -> MATLAB Function1/5(plane_DA)
  Demux3/2 -> MATLAB Function1/3(plane_BC)
  Sum2/1 -> Quantizer/1
  Demux3/3 -> MATLAB Function1/4(plane_CD)
  AHRS Pitch/1 -> MATLAB Function1/8(Pitch)
  Demux3/1 -> MATLAB Function1/2(plane_AB)
  AHRS Roll/1 -> MATLAB Function1/7(Roll)
  AHRS Yaw/1 -> MATLAB Function1/9(Yaw)
  " WN Sonar DX "/1 -> Sum2/2
  LAT-LON/1 -> MATLAB Function1/1(pos)
  Demux3/5 -> MATLAB Function1/6(plane_W)

== system sim_all/Sensors/Environment and Sensors Model4 ==
  LAT-LON : Inport  SampleTime=sens_Sample_time_sonar
  Environment : Inport  Port=2  SampleTime=sens_Sample_time_sonar
  AHRS Roll : Inport  Port=3  SampleTime=sens_Sample_time_sonar
  AHRS Pitch : Inport  Port=4  SampleTime=sens_Sample_time_sonar
  AHRS Yaw : Inport  Port=5  SampleTime=sens_Sample_time_sonar
  " WN Sonar SX " : RandomNumber  Variance=sens_Variance_sonar  Seed=4321  SampleTime=sens_Sample_time_sonar
  Constant : Constant  Value=sens_distCM
  Demux3 : Demux  Outputs=5
  MATLAB Function1 : MATLAB Function  TreatAsAtomicUnit=on
  Quantizer : Quantizer  QuantizationInterval=sens_Resolution_sonar  LinearizeAsGain=off
  Sum1 : Sum  Inputs=|+-
  Sum2 : Sum  Inputs=|++
  Sonar SX : Outport
  wires:
  MATLAB Function1/1(dist) -> Sum1/1
  Sum1/1 -> Sum2/1
  Constant/1 -> Sum1/2
  Environment/1 -> Demux3/1
  Quantizer/1 -> Sonar SX/1
  Demux3/4 -> MATLAB Function1/5(plane_DA)
  Demux3/2 -> MATLAB Function1/3(plane_BC)
  Sum2/1 -> Quantizer/1
  Demux3/3 -> MATLAB Function1/4(plane_CD)
  AHRS Pitch/1 -> MATLAB Function1/8(Pitch)
  Demux3/1 -> MATLAB Function1/2(plane_AB)
  AHRS Roll/1 -> MATLAB Function1/7(Roll)
  AHRS Yaw/1 -> MATLAB Function1/9(Yaw)
  " WN Sonar SX "/1 -> Sum2/2
  LAT-LON/1 -> MATLAB Function1/1(pos)
  Demux3/5 -> MATLAB Function1/6(plane_W)

== system sim_all/Sensors/Environment and Sensors Model6 ==
  LAT-LON : Inport  SampleTime=sens_Sample_time_sonar
  Environment : Inport  Port=2  SampleTime=sens_Sample_time_sonar
  AHRS Roll : Inport  Port=3  SampleTime=sens_Sample_time_sonar
  AHRS Pitch : Inport  Port=4  SampleTime=sens_Sample_time_sonar
  AHRS Yaw : Inport  Port=5  SampleTime=sens_Sample_time_sonar
  " WN Sonar Prua " : RandomNumber  Variance=sens_Variance_sonar  Seed=1234  SampleTime=sens_Sample_time_sonar
  Constant : Constant  Value=sens_distCM
  Demux3 : Demux  Outputs=5
  MATLAB Function1 : MATLAB Function  TreatAsAtomicUnit=on
  Quantizer : Quantizer  QuantizationInterval=sens_Resolution_sonar  LinearizeAsGain=off
  Sum1 : Sum  Inputs=|+-
  Sum2 : Sum  Inputs=|++
  Sonar Prua : Outport
  wires:
  Demux3/3 -> MATLAB Function1/4(plane_CD)
  " WN Sonar Prua "/1 -> Sum2/2
  LAT-LON/1 -> MATLAB Function1/1(pos)
  Demux3/1 -> MATLAB Function1/2(plane_AB)
  Demux3/4 -> MATLAB Function1/5(plane_DA)
  Sum2/1 -> Quantizer/1
  Demux3/2 -> MATLAB Function1/3(plane_BC)
  Quantizer/1 -> Sonar Prua/1
  Environment/1 -> Demux3/1
  AHRS Roll/1 -> MATLAB Function1/7(Roll)
  AHRS Pitch/1 -> MATLAB Function1/8(Pitch)
  AHRS Yaw/1 -> MATLAB Function1/9(Yaw)
  MATLAB Function1/1(dist) -> Sum1/1
  Sum1/1 -> Sum2/1
  Constant/1 -> Sum1/2
  Demux3/5 -> MATLAB Function1/6(plane_W)

== system sim_all/Controller_mk4_v3/C_or/C_va_X_td ==
  err_va : Inport
  Reset : ResetPort  DisableCoverage=on
  LTI System : cstblocks/LTI System  sys=ctrl_Cva_td3  IC=[]
  tau : Outport
  wires:
  err_va/1 -> LTI System/1
  LTI System/1 -> tau/1

== system sim_all/Controller_mk4_v3/C_or/C_va_Y_td ==
  err_va : Inport
  Reset : ResetPort  DisableCoverage=on
  LTI System : cstblocks/LTI System  sys=ctrl_Cva_td3  IC=[]
  tau : Outport
  wires:
  LTI System/1 -> tau/1
  err_va/1 -> LTI System/1

== system sim_all/Controller_mk4_v3/C_or/C_va_Z_td ==
  err_va : Inport
  Reset : ResetPort  DisableCoverage=on
  LTI System : cstblocks/LTI System  sys=ctrl_Cva_td3  IC=[]
  tau : Outport
  wires:
  err_va/1 -> LTI System/1
  LTI System/1 -> tau/1

== system sim_all/Controller_mk4_v3/C_pos/abs_integrator1 ==
  err_x : Inport
  err_y : Inport  Port=2
  err_z : Inport  Port=3
  enabler : Inport  Port=4
  Body2Ned : MATLAB Function  TreatAsAtomicUnit=on
  Demux : Demux  Outputs=3
  Discrete-Time Integrator : DiscreteIntegrator  gainval=ctrl_Ki_pos  ExternalReset=rising  SampleTime=ctrl_Ts  ICPrevOutput=DiscIntNeverNeededParam  ICPrevScaledInput=DiscIntNeverNeededParam
  Mux : Mux  Inputs=3
  Ned2Body1 : MATLAB Function  TreatAsAtomicUnit=on
  int_x : Outport
  int_y : Outport  Port=2
  int_z : Outport  Port=3
  wires:
  [Or] -> Ned2Body1/2(or), Body2Ned/2(or)
  enabler/1 -> Discrete-Time Integrator/2
  Body2Ned/1(x_n) -> Discrete-Time Integrator/1
  err_x/1 -> Mux/1
  err_y/1 -> Mux/2
  Mux/1 -> Body2Ned/1(x_b)
  Ned2Body1/1(x_b) -> Demux/1
  Demux/1 -> int_x/1
  Demux/2 -> int_y/1
  Demux/3 -> int_z/1
  err_z/1 -> Mux/3
  Discrete-Time Integrator/1 -> Ned2Body1/1(x_n)

== system sim_all/Controller_mk4_v3/C_pos/abs_integrator2 ==
  err_vx : Inport
  err_vy : Inport  Port=2
  err_vz : Inport  Port=3
  enabler : Inport  Port=4
  Body2Ned : MATLAB Function  TreatAsAtomicUnit=on
  Demux : Demux  Outputs=3
  Discrete-Time Integrator : DiscreteIntegrator  gainval=ctrl_Ki_v_pos  ExternalReset=rising  SampleTime=ctrl_Ts  ICPrevOutput=DiscIntNeverNeededParam  ICPrevScaledInput=DiscIntNeverNeededParam
  Mux : Mux  Inputs=3
  Ned2Body1 : MATLAB Function  TreatAsAtomicUnit=on
  int_vx : Outport
  int_vy : Outport  Port=2
  int_vz : Outport  Port=3
  wires:
  Demux/3 -> int_vz/1
  Demux/2 -> int_vy/1
  Demux/1 -> int_vx/1
  Ned2Body1/1(x_b) -> Demux/1
  Mux/1 -> Body2Ned/1(x_b)
  err_vy/1 -> Mux/2
  err_vx/1 -> Mux/1
  [Or] -> Body2Ned/2(or), Ned2Body1/2(or)
  err_vz/1 -> Mux/3
  Body2Ned/1(x_n) -> Discrete-Time Integrator/1
  enabler/1 -> Discrete-Time Integrator/2
  Discrete-Time Integrator/1 -> Ned2Body1/1(x_n)

== system sim_all/Controller_mk4_v3/C_vel/abs_integrator ==
  err_vx : Inport
  err_vy : Inport  Port=2
  err_vz : Inport  Port=3
  enabler : Inport  Port=4
  Body2Ned : MATLAB Function  TreatAsAtomicUnit=on
  Demux : Demux  Outputs=3
  Discrete-Time Integrator : DiscreteIntegrator  gainval=ctrl_Ki_vel  ExternalReset=rising  SampleTime=ctrl_Ts  ICPrevOutput=DiscIntNeverNeededParam  ICPrevScaledInput=DiscIntNeverNeededParam
  Mux : Mux  Inputs=3
  Ned2Body1 : MATLAB Function  TreatAsAtomicUnit=on
  int_vx : Outport
  int_vy : Outport  Port=2
  int_vz : Outport  Port=3
  wires:
  Demux/3 -> int_vz/1
  Demux/2 -> int_vy/1
  Demux/1 -> int_vx/1
  Ned2Body1/1(x_b) -> Demux/1
  Mux/1 -> Body2Ned/1(x_b)
  err_vy/1 -> Mux/2
  err_vx/1 -> Mux/1
  [Or] -> Body2Ned/2(or), Ned2Body1/2(or)
  err_vz/1 -> Mux/3
  Body2Ned/1(x_n) -> Discrete-Time Integrator/1
  enabler/1 -> Discrete-Time Integrator/2
  Discrete-Time Integrator/1 -> Ned2Body1/1(x_n)

== system sim_all/Controller_mk4_v3/signal_to_NED/Signal_d->NED ==
  Vel_d : Inport
  Dpp_d : Inport  Port=2
  Dps_d : Inport  Port=3
  Orp_d : Inport  Port=4
  Wall : Inport  Port=5
  ToNed : MATLAB Function  TreatAsAtomicUnit=on
  wall_fcn : MATLAB Function  TreatAsAtomicUnit=on
  Vel_d_ned : Outport  VectorParamsAs1DForOutWhenUnconnected=off
  Dpp_d_ned : Outport  Port=2  VectorParamsAs1DForOutWhenUnconnected=off
  Dps_d_ned : Outport  Port=3  VectorParamsAs1DForOutWhenUnconnected=off
  Orp_d_ned : Outport  Port=4  VectorParamsAs1DForOutWhenUnconnected=off
  wires:
  wall_fcn/1(wall_vect) -> ToNed/5(wall_vect)
  ToNed/3(dps_n) -> Dps_d_ned/1
  Wall/1 -> wall_fcn/1(WALL)
  Dpp_d/1 -> ToNed/2(ddp)
  ToNed/2(ddp_n) -> Dpp_d_ned/1
  ToNed/1(vel_n) -> Vel_d_ned/1
  Orp_d/1 -> ToNed/4(orp)
  ToNed/4(orp_n) -> Orp_d_ned/1
  Dps_d/1 -> ToNed/3(dps)
  Vel_d/1 -> ToNed/1(vel)
  wall_fcn/2(wall_vect2) -> ToNed/6(wall_vect2)
  [current_state] -> ToNed/7(state)

== system sim_all/Controller_mk4_v3/signal_to_NED/Signal_s->NED ==
  Dpp_s : Inport
  Dps_s : Inport  Port=2
  Wall : Inport  Port=3
  ToNed : MATLAB Function  TreatAsAtomicUnit=on
  wall_fcn1 : MATLAB Function  TreatAsAtomicUnit=on
  Dpp_s_ned : Outport  VectorParamsAs1DForOutWhenUnconnected=off
  Dps_s_ned : Outport  Port=2  VectorParamsAs1DForOutWhenUnconnected=off
  wires:
  Dpp_s/1 -> ToNed/1(ddp)
  ToNed/1(ddp_n) -> Dpp_s_ned/1
  Dps_s/1 -> ToNed/2(dps)
  ToNed/2(dps_n) -> Dps_s_ned/1
  Wall/1 -> wall_fcn1/1(WALL)
  wall_fcn1/1(wall_vect) -> ToNed/3(wall_vect)
  wall_fcn1/2(wall_vect2) -> ToNed/4(wall_vect2)

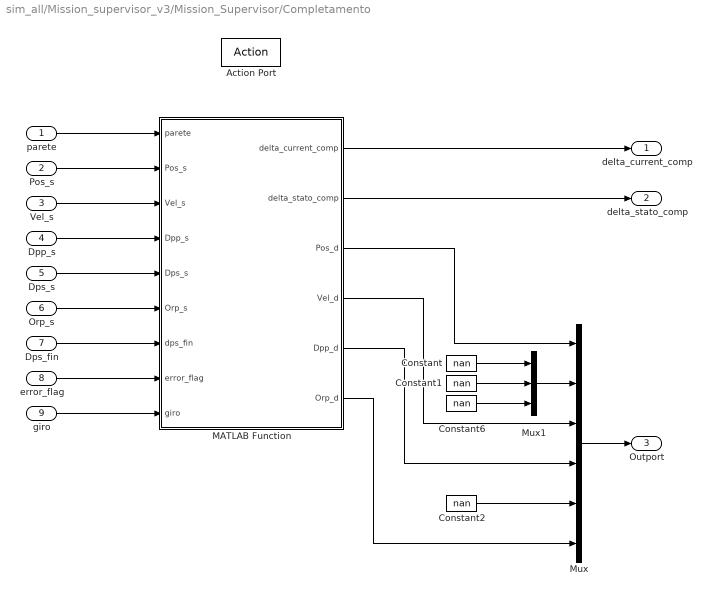
== system sim_all/Mission_supervisor_v3/Mission_Supervisor/Completamento ==
  parete : Inport
  Pos_s : Inport  Port=2
  Vel_s : Inport  Port=3
  Dpp_s : Inport  Port=4
  Dps_s : Inport  Port=5
  Orp_s : Inport  Port=6
  Dps_fin : Inport  Port=7
  error_flag : Inport  Port=8
  giro : Inport  Port=9
  Action Port : ActionPort  ActionPortLabel=case [ 204 ]:
  Constant{,1..2,6} (4 alike) : Constant  Value=nan
  MATLAB Function : MATLAB Function  TreatAsAtomicUnit=on  SystemSampleTime=Ts_supervisor
  Mux : Mux  Inputs=6
  Mux1 : Mux  Inputs=3
  delta_current_comp : Outport
  delta_stato_comp : Outport  Port=2
  Outport : Outport  Port=3
  wires:
  MATLAB Function/1(delta_current_comp) -> delta_current_comp/1
  MATLAB Function/2(delta_stato_comp) -> delta_stato_comp/1
  parete/1 -> MATLAB Function/1(parete)
  MATLAB Function/3(Pos_d) -> Mux/1
  Mux/1 -> Outport/1
  MATLAB Function/4(Vel_d) -> Mux/3
  MATLAB Function/5(Dpp_d) -> Mux/4
  MATLAB Function/6(Orp_d) -> Mux/6
  Constant/1 -> Mux1/1
  Constant1/1 -> Mux1/2
  Constant6/1 -> Mux1/3
  Mux1/1 -> Mux/2
  Constant2/1 -> Mux/5
  Pos_s/1 -> MATLAB Function/2(Pos_s)
  Vel_s/1 -> MATLAB Function/3(Vel_s)
  Dpp_s/1 -> MATLAB Function/4(Dpp_s)
  Dps_s/1 -> MATLAB Function/5(Dps_s)
  Orp_s/1 -> MATLAB Function/6(Orp_s)
  Dps_fin/1 -> MATLAB Function/7(dps_fin)
  error_flag/1 -> MATLAB Function/8(error_flag)
  giro/1 -> MATLAB Function/9(giro)

== system sim_all/Mission_supervisor_v3/Mission_Supervisor/Fine missione ==
  current_state : Inport
  Action Port : ActionPort  ActionPortLabel=case [ 304 ]:
  Constant{1..7} (7 alike) : Constant  Value=nan
  MATLAB Function : MATLAB Function  TreatAsAtomicUnit=on  SystemSampleTime=Ts_supervisor
  Mux : Mux  Inputs=6
  Mux1 : Mux  Inputs=3
  delta_current_end : Outport
  Outport : Outport  Port=2
  wires:
  MATLAB Function/1(delta_current_end) -> delta_current_end/1
  current_state/1 -> MATLAB Function/1(stato)
  Mux/1 -> Outport/1
  Constant2/1 -> Mux/3
  Constant3/1 -> Mux/4
  Constant4/1 -> Mux/5
  Constant5/1 -> Mux/6
  Constant1/1 -> Mux1/1
  Constant6/1 -> Mux1/2
  Constant7/1 -> Mux1/3
  Mux1/1 -> Mux/1, Mux/2

== system sim_all/Mission_supervisor_v3/Mission_Supervisor/Frenata in completamento ==
  Pos_s : Inport
  Orp_s : Inport  Port=2
  Dpp_s : Inport  Port=3
  Dps_s : Inport  Port=4
  dps_fin : Inport  Port=5
  error_flag : Inport  Port=6
  Action Port : ActionPort  ActionPortLabel=case [ 205 ]:
  Constant{,1..2,6} (4 alike) : Constant  Value=nan
  MATLAB Function : MATLAB Function  TreatAsAtomicUnit=on  SystemSampleTime=Ts_supervisor
  Mux : Mux  Inputs=6
  Mux1 : Mux  Inputs=3
  delta_current_fren_comp : Outport
  delta_stato_fren_comp : Outport  Port=2
  SOS_205 : Outport  Port=3
  " " : Outport  Port=4
  wires:
  MATLAB Function/1(delta_current_fren_comp) -> delta_current_fren_comp/1
  MATLAB Function/2(delta_stato_fren_comp) -> delta_stato_fren_comp/1
  MATLAB Function/4(Pos_d) -> Mux/1
  MATLAB Function/5(Dpp_d) -> Mux/4
  MATLAB Function/6(Dps_d) -> Mux/5
  MATLAB Function/7(Orp_d) -> Mux/6
  Constant/1 -> Mux1/1
  Constant1/1 -> Mux1/2
  Constant6/1 -> Mux1/3
  Mux1/1 -> Mux/2
  Constant2/1 -> Mux/3
  Pos_s/1 -> MATLAB Function/1(Pos_s)
  Orp_s/1 -> MATLAB Function/2(Orp_s)
  Dpp_s/1 -> MATLAB Function/3(Dpp_s)
  Dps_s/1 -> MATLAB Function/4(Dps_s)
  dps_fin/1 -> MATLAB Function/5(dps_fin)
  error_flag/1 -> MATLAB Function/6(error_flag)
  MATLAB Function/3(SOS_205) -> SOS_205/1
  Mux/1 -> " "/1

== system sim_all/Mission_supervisor_v3/Mission_Supervisor/Frenata pattugliamento ==
  contatore : Inport
  Pos_s : Inport  Port=2
  Dpp_s : Inport  Port=3
  Dps_s : Inport  Port=4
  Orp_s : Inport  Port=5
  error_flag : Inport  Port=6
  Action Port : ActionPort  ActionPortLabel=case [ 202 ]:
  Constant{,1..2,6} (4 alike) : Constant  Value=nan
  MATLAB Function : MATLAB Function  TreatAsAtomicUnit=on  SystemSampleTime=Ts_supervisor
  Mux : Mux  Inputs=6
  Mux1 : Mux  Inputs=3
  delta_current_fren_patt : Outport
  delta_stato_fren_patt : Outport  Port=2
  Outport : Outport  Port=3
  wires:
  MATLAB Function/1(delta_current_fren_patt) -> delta_current_fren_patt/1
  MATLAB Function/2(delta_stato_fren_patt) -> delta_stato_fren_patt/1
  MATLAB Function/3(Pos_d) -> Mux/1
  Mux/1 -> Outport/1
  contatore/1 -> MATLAB Function/1(contatore)
  MATLAB Function/4(Dpp_d) -> Mux/4
  MATLAB Function/5(Dps_d) -> Mux/5
  MATLAB Function/6(Orp_d) -> Mux/6
  Constant/1 -> Mux1/1
  Constant1/1 -> Mux1/2
  Constant6/1 -> Mux1/3
  Mux1/1 -> Mux/2
  Constant2/1 -> Mux/3
  Pos_s/1 -> MATLAB Function/2(Pos_s)
  Dpp_s/1 -> MATLAB Function/3(Dpp_s)
  Dps_s/1 -> MATLAB Function/4(Dps_s)
  Orp_s/1 -> MATLAB Function/5(Orp_s)
  error_flag/1 -> MATLAB Function/6(error_flag)

== system sim_all/Mission_supervisor_v3/Mission_Supervisor/Immersione ==
  Pos_s : Inport
  punto_iniz_patt : Inport  Port=2
  Or_in : Inport  Port=3
  error_flag : Inport  Port=4
  Action Port : ActionPort  ActionPortLabel=case [ 103 ]:
  Constant{,1..3} (4 alike) : Constant  Value=nan
  MATLAB Function : MATLAB Function  TreatAsAtomicUnit=on  SystemSampleTime=Ts_supervisor
  Mux : Mux  Inputs=6
  delta_current_immers : Outport
  delta_stato_immers : Outport  Port=2
  Outport : Outport  Port=3
  wires:
  MATLAB Function/1(delta_current_immers) -> delta_current_immers/1
  MATLAB Function/2(delta_stato_immers) -> delta_stato_immers/1
  MATLAB Function/3(Pos_d) -> Mux/1
  Mux/1 -> Outport/1
  Constant/1 -> Mux/3
  Constant1/1 -> Mux/6
  Constant2/1 -> Mux/5
  Pos_s/1 -> MATLAB Function/1(Pos_s)
  punto_iniz_patt/1 -> MATLAB Function/2(punto_iniz_patt)
  error_flag/1 -> MATLAB Function/4(error_flag)
  MATLAB Function/4(Or_d) -> Mux/2
  Or_in/1 -> MATLAB Function/3(Or_in)
  Constant3/1 -> Mux/4

== system sim_all/Mission_supervisor_v3/Mission_Supervisor/Inizio ==
  Pos_s : Inport
  error_flag : Inport  Port=2
  Action Port : ActionPort  ActionPortLabel=case [ 100 ]:
  Constant{,1..5,7} (7 alike) : Constant  Value=nan
  Digital Clock : DigitalClock  SampleTime=0.1
  MATLAB Function : MATLAB Function  TreatAsAtomicUnit=on  SystemSampleTime=Ts_supervisor
  Mux : Mux  Inputs=6
  Mux1 : Mux  Inputs=3
  current_state : Outport
  parete_attuale : Outport  Port=2
  delta_stato : Outport  Port=3
  Outport : Outport  Port=4
  wires:
  MATLAB Function/1(current_state) -> current_state/1
  MATLAB Function/2(parete_attuale) -> parete_attuale/1
  MATLAB Function/3(stato_interno) -> delta_stato/1
  Mux/1 -> Outport/1
  Mux1/1 -> Mux/2
  Constant2/1 -> Mux/3
  Constant3/1 -> Mux/4
  Constant4/1 -> Mux/5
  Constant5/1 -> Mux/6
  Constant/1 -> Mux1/1
  Constant7/1 -> Mux1/2
  Constant1/1 -> Mux1/3
  Pos_s/1 -> MATLAB Function/1(Pos_s)
  MATLAB Function/4(Pos_d) -> Mux/1
  Digital Clock/1 -> MATLAB Function/3(attesa)
  error_flag/1 -> MATLAB Function/2(error_flag)

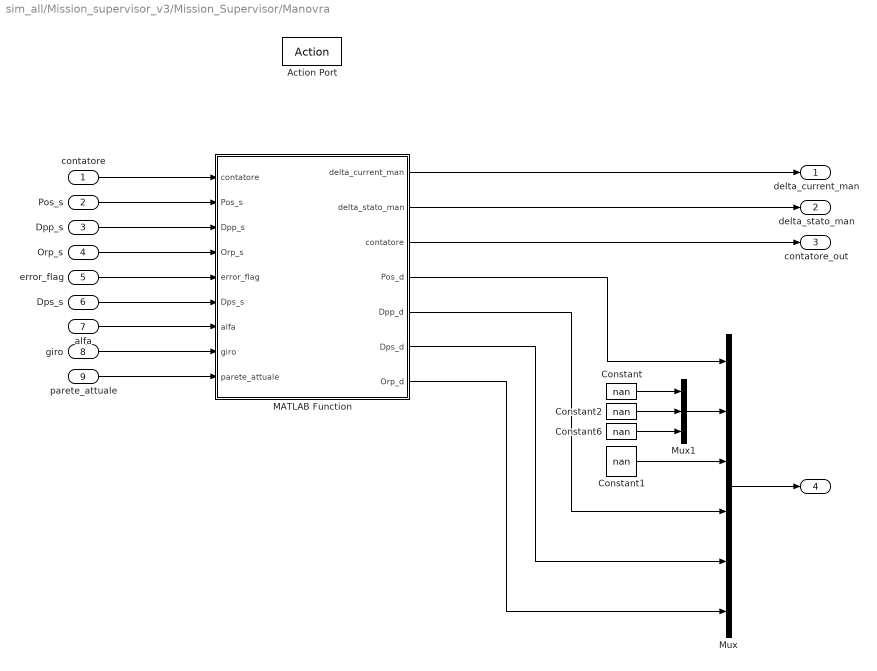
== system sim_all/Mission_supervisor_v3/Mission_Supervisor/Manovra ==
  contatore : Inport
  Pos_s : Inport  Port=2
  Dpp_s : Inport  Port=3
  Orp_s : Inport  Port=4
  error_flag : Inport  Port=5
  Dps_s : Inport  Port=6
  alfa : Inport  Port=7
  giro : Inport  Port=8
  parete_attuale : Inport  Port=9
  Action Port : ActionPort  ActionPortLabel=case [ 203 ]:
  Constant{,1..2,6} (4 alike) : Constant  Value=nan
  MATLAB Function : MATLAB Function  TreatAsAtomicUnit=on  SystemSampleTime=Ts_supervisor
  Mux : Mux  Inputs=6
  Mux1 : Mux  Inputs=3
  delta_current_man : Outport
  delta_stato_man : Outport  Port=2
  contatore_out : Outport  Port=3
  "  " : Outport  Port=4
  wires:
  MATLAB Function/1(delta_current_man) -> delta_current_man/1
  MATLAB Function/2(delta_stato_man) -> delta_stato_man/1
  contatore/1 -> MATLAB Function/1("contatore ")
  MATLAB Function/4(Pos_d) -> Mux/1
  Constant1/1 -> Mux/3
  MATLAB Function/5(Dpp_d) -> Mux/4
  MATLAB Function/6(Dps_d) -> Mux/5
  MATLAB Function/7(Orp_d) -> Mux/6
  Constant/1 -> Mux1/1
  Constant2/1 -> Mux1/2
  Constant6/1 -> Mux1/3
  Mux1/1 -> Mux/2
  Pos_s/1 -> MATLAB Function/2(Pos_s)
  Dpp_s/1 -> MATLAB Function/3(Dpp_s)
  Orp_s/1 -> MATLAB Function/4(Orp_s)
  error_flag/1 -> MATLAB Function/5(error_flag)
  Dps_s/1 -> MATLAB Function/6(Dps_s)
  MATLAB Function/3(contatore) -> contatore_out/1
  Mux/1 -> "  "/1
  alfa/1 -> MATLAB Function/7(alfa)
  giro/1 -> MATLAB Function/8(giro)
  parete_attuale/1 -> MATLAB Function/9(parete_attuale)
